simulink model "s12_euler_fvm_periodic_step_muscl_minmod_ref"  (R2026a)
settings: Solver=FixedStepDiscrete  StopTime=0
model workspace (MAT data in the model file):
  S12_FVM_CFL = Simulink.Parameter
  S12_FVM_CFL.Value = 0.45
  S12_FVM_CFL.Complexity = 'real'
  S12_FVM_CFL.Dimensions = [1 1]
  S12_FVM_CFL.Description = 'Maximum CFL number'
  S12_FVM_CFL.DataType = 'auto'
  S12_FVM_DtRequest = Simulink.Parameter
  S12_FVM_DtRequest.Value = 0.001
  S12_FVM_DtRequest.Complexity = 'real'
  S12_FVM_DtRequest.Dimensions = [1 1]
  S12_FVM_DtRequest.Description = 'Requested explicit time step'
  S12_FVM_DtRequest.DataType = 'auto'
  S12_FVM_Dx = Simulink.Parameter
  S12_FVM_Dx.Value = 0.01
  S12_FVM_Dx.Complexity = 'real'
  S12_FVM_Dx.Dimensions = [1 1]
  S12_FVM_Dx.Description = 'Uniform cell length'
  S12_FVM_Dx.DataType = 'auto'
  S12_FVM_Gamma = Simulink.Parameter
  S12_FVM_Gamma.Value = 1.4
  S12_FVM_Gamma.Complexity = 'real'
  S12_FVM_Gamma.Dimensions = [1 1]
  S12_FVM_Gamma.Description = 'Heat capacity ratio'
  S12_FVM_Gamma.DataType = 'auto'
  S12_FVM_State = Simulink.Parameter
  S12_FVM_State.Value = [1  1  1  1  0.125  0.125  0.125  0.125; 0  0  0  0  0  0  0  0; 250000  250000  250000  250000  25000  25000  25000  25000]
  S12_FVM_State.Complexity = 'real'
  S12_FVM_State.Dimensions = [3 8]
  S12_FVM_State.Description = 'Rows: density, momentum density, total energy density'
  S12_FVM_State.DataType = 'auto'
settings Model: Creator=Jovi  LastModifiedBy=Jovi

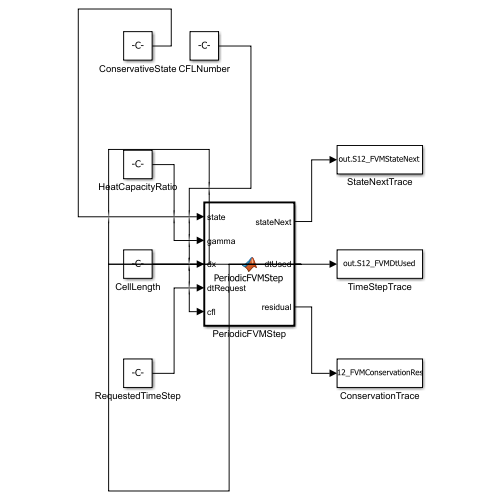
[thumbnail: Simulink's stored preview of the top-level diagram]
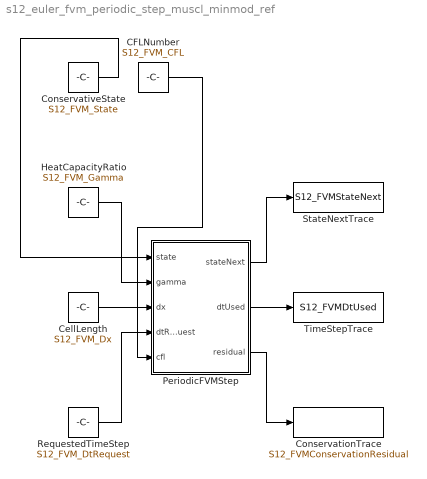
== system s12_euler_fvm_periodic_step_muscl_minmod_ref ==
  CFLNumber : Constant  Value=S12_FVM_CFL
  CellLength : Constant  Value=S12_FVM_Dx
  ConservationTrace : ToWorkspace  VariableName=S12_FVMConservationResidual
      settings: MaxDataPoints=100
  ConservativeState : Constant  Value=S12_FVM_State
  HeatCapacityRatio : Constant  Value=S12_FVM_Gamma
  PeriodicFVMStep : MATLAB Function  TreatAsAtomicUnit=on
  RequestedTimeStep : Constant  Value=S12_FVM_DtRequest
  StateNextTrace : ToWorkspace  VariableName=S12_FVMStateNext
      settings: MaxDataPoints=100
  TimeStepTrace : ToWorkspace  VariableName=S12_FVMDtUsed
      settings: MaxDataPoints=100
  wires:
  ConservativeState/1 -> PeriodicFVMStep/1(state)
  HeatCapacityRatio/1 -> PeriodicFVMStep/2(gamma)
  CellLength/1 -> PeriodicFVMStep/3(dx)
  RequestedTimeStep/1 -> PeriodicFVMStep/4(dtRequest)
  CFLNumber/1 -> PeriodicFVMStep/5(cfl)
  PeriodicFVMStep/1(stateNext) -> StateNextTrace/1
  PeriodicFVMStep/2(dtUsed) -> TimeStepTrace/1
  PeriodicFVMStep/3(residual) -> ConservationTrace/1

== matlab function s12_euler_fvm_periodic_step_muscl_minmod_ref/PeriodicFVMStep ==
  data: state input; stateNext output; gamma input; dx input; dtRequest input; cfl input; dtUsed output; residual output
function [stateNext,dtUsed,residual] = PeriodicFVMStep(state,gamma,dx,dtRequest,cfl)
%#codegen
cellCount = size(state,2);
interfaceFlux = zeros(3,cellCount);
maxSignalSpeed = 0;
for cellIndex = 1:cellCount
    density = state(1,cellIndex);
    velocity = state(2,cellIndex)/density;
    pressure = (gamma-1)*(state(3,cellIndex)-0.5*density*velocity*velocity);
    soundSpeed = sqrt(gamma*pressure/density);
    maxSignalSpeed = max(maxSignalSpeed,abs(velocity)+soundSpeed);
end
dtUsed = min(dtRequest,cfl*dx/maxSignalSpeed);
[rho,velocity,pressure] = recoverPrimitives(state,gamma);
slopeRho = minmodSlopes(rho);
slopeVelocity = minmodSlopes(velocity);
slopePressure = minmodSlopes(pressure);
for interfaceIndex = 1:cellCount
    rightIndex = interfaceIndex+1;
    if rightIndex > cellCount
        rightIndex = 1;
    end
    leftState = conservativeFromPrimitives(rho(interfaceIndex) + 0.5*slopeRho(interfaceIndex),velocity(interfaceIndex) + 0.5*slopeVelocity(interfaceIndex),pressure(interfaceIndex) + 0.5*slopePressure(interfaceIndex),gamma);
    rightState = conservativeFromPrimitives(rho(rightIndex) - 0.5*slopeRho(rightIndex),velocity(rightIndex) - 0.5*slopeVelocity(rightIndex),pressure(rightIndex) - 0.5*slopePressure(rightIndex),gamma);
    interfaceFlux(:,interfaceIndex) = hllcFlux(leftState,rightState,gamma);
end
stateNext = zeros(size(state));
for cellIndex = 1:cellCount
    leftInterface = cellIndex-1;
    if leftInterface < 1
        leftInterface = cellCount;
    end
    stateNext(:,cellIndex) = state(:,cellIndex) - dtUsed/dx*(interfaceFlux(:,cellIndex)-interfaceFlux(:,leftInterface));
end
residual = sum(stateNext-state,2).';
end

function flux = hllcFlux(stateL,stateR,gamma)
rhoL = stateL(1);
rhoR = stateR(1);
uL = stateL(2)/rhoL;
uR = stateR(2)/rhoR;
energyL = stateL(3);
energyR = stateR(3);
pL = (gamma-1)*(energyL-0.5*rhoL*uL*uL);
pR = (gamma-1)*(energyR-0.5*rhoR*uR*uR);
soundL = sqrt(gamma*pL/rhoL);
soundR = sqrt(gamma*pR/rhoR);
sL = min(uL-soundL,uR-soundR);
sR = max(uL+soundL,uR+soundR);
denominator = rhoL*(sL-uL)-rhoR*(sR-uR);
sM = (pR-pL+rhoL*uL*(sL-uL)-rhoR*uR*(sR-uR))/denominator;
fluxL = [rhoL*uL;rhoL*uL*uL+pL;uL*(energyL+pL)];
fluxR = [rhoR*uR;rhoR*uR*uR+pR;uR*(energyR+pR)];
if sL >= 0
    flux = fluxL;
elseif sM >= 0
    rhoStarL = rhoL*(sL-uL)/(sL-sM);
    energyStarL = rhoStarL*(energyL/rhoL+(sM-uL)*(sM+pL/(rhoL*(sL-uL))));
    stateStarL = [rhoStarL;rhoStarL*sM;energyStarL];
    flux = fluxL+sL*(stateStarL-stateL);
elseif sR > 0
    rhoStarR = rhoR*(sR-uR)/(sR-sM);
    energyStarR = rhoStarR*(energyR/rhoR+(sM-uR)*(sM+pR/(rhoR*(sR-uR))));
    stateStarR = [rhoStarR;rhoStarR*sM;energyStarR];
    flux = fluxR+sR*(stateStarR-stateR);
else
    flux = fluxR;
end
end
function [rho,velocity,pressure] = recoverPrimitives(state,gamma)
rho = state(1,:);
velocity = state(2,:)./rho;
pressure = (gamma-1)*(state(3,:) - 0.5*rho.*velocity.^2);
end

function state = conservativeFromPrimitives(rho,velocity,pressure,gamma)
state = [rho; rho.*velocity; pressure/(gamma-1) + 0.5*rho.*velocity.^2];
end

function slopes = minmodSlopes(values)
cellCount = numel(values);
slopes = zeros(size(values));
if cellCount < 3
    return
end
for cellIndex = 1:cellCount
    leftIndex = cellIndex - 1;
    if leftIndex < 1
        leftIndex = cellCount;
    end
    rightIndex = cellIndex + 1;
    if rightIndex > cellCount
        rightIndex = 1;
    end
    slopes(cellIndex) = minmod(values(cellIndex)-values(leftIndex),values(rightIndex)-values(cellIndex));
end
end

function value = minmod(leftDelta,rightDelta)
if leftDelta*rightDelta <= 0
    value = 0;
elseif abs(leftDelta) <= abs(rightDelta)
    value = leftDelta;
else
    value = rightDelta;
end
end
